simulink model "hyd_hyb_2_sec_con_1"  (Simulink 7.7)
settings: Solver=ode14x  StartTime=0  StopTime=994  FixedStep=0.01  MaxStep=.4  RelTol=1e-8
InitFcn:
  | const_3
values from neighbouring files (symbols this model uses):
  Af = 6.3    [brk_enrg.m]    (also in brk_enrg_1.m)
  BSFC_906_205 = [3.5684 4.3466 5.1668 6.0769 6.988 7.8992 8.8104 9.7336 10.8548 11.9809 13.1112 14.2571 ... (663 elements, 39x17)]    [BSFC_map_906_205.mat]
  Cd = 0.55    [brk_enrg.m]    (also in brk_enrg_1.m)
  den = 1.202    [brk_enrg.m]    (also in brk_enrg_1.m)
  fr = 0.01    [brk_enrg.m]    (also in brk_enrg_1.m)
undefined symbols (not defined in the file or in its folder): clutchRise, down_spd_2, down_spd_3, down_spd_4, down_spd_c, fuel_density, gearshift, I_wheel, Idle_spd_eng_906, M1_hydr, p_v_15, pmax_125, qv_125, Rw, sec_eng_sfc_map, soc_1, soc_2, T_0, T_1, T_2, T_max_906, T_min, t_wait_1, t_wait_2, t_wait_3, TC_spd_ratio_max, torque_convertor, Twait, up_spd_1, up_spd_2, up_spd_3, up_spd_c, v_p_10, v_p_15, v_p_5, veh_spd_0
libraries: fl_lib x43, nesl_utility x30, sdl_lib x14, simulink x5, simulink_need_slupdate x1
(part 3 of 3)

== system hyd_hyb_2_sec_con_1/hydraulic transmission/accumulator/max - min volume estimator/for 10 gal accumulator ==
  min_press(psi) : Inport
  max_press(psi) : Inport  Port=2
  pre_ch_press(psi) : Inport  Port=3
  Action Port : ActionPort  PropagateVarSize=During execution  ActionType=then
  Constant : Constant  Value=152
  Scope : Scope  NumInputPorts=2
      settings: YMin=-5~-5  YMax=5~5  SaveName=ScopeData40
  Scope1 : Scope  NumInputPorts=2
      settings: YMin=-5~-5  YMax=5~5  SaveName=ScopeData41
  in^3 to lit : Gain  Gain=16.387e-3
  in^3 to lit (1) : Gain  Gain=16.387e-3
  rexroth-1 : Lookup_n-D  BreakpointsForDimension1=[1000,1100,1200,1300,1400,1500,1600,1700,1800,1900,2000,2100,2200,2300,2400,2500,2600,2700,2800,2900,3000,3100,3200,3300,3400,3500,3600,3700,3800,3900,4000,4100,4200,4300,4400,4500,4600,4700,4800,4900,5000,5100,5200,5300,5400,5500,5600,5700,5800,5900,6000]  BreakpointsForDimension2=[1000,1400,2000]  Table=v_p_10  InputSameDT=on
  rexroth-10 : Lookup_n-D  BreakpointsForDimension1=[1000,1100,1200,1300,1400,1500,1600,1700,1800,1900,2000,2100,2200,2300,2400,2500,2600,2700,2800,2900,3000,3100,3200,3300,3400,3500,3600,3700,3800,3900,4000,4100,4200,4300,4400,4500,4600,4700,4800,4900,5000,5100,5200,5300,5400,5500,5600,5700,5800,5900,6000]  BreakpointsForDimension2=[1000,1400,2000]  Table=v_p_10  InputSameDT=on
  min_vol(lit) : Outport
  max_vol(lit) : Outport  Port=2
  accum_dry_mass ( kg ) : Outport  Port=3  InitialOutput=[0]
  wires:
  in^3 to lit/1 -> min_vol(lit)/1, Scope1/1
  rexroth-10/1 -> in^3 to lit (1)/1, Scope/2
  rexroth-1/1 -> in^3 to lit/1, Scope/1
  in^3 to lit (1)/1 -> max_vol(lit)/1, Scope1/2
  pre_ch_press(psi)/1 -> rexroth-10/2, rexroth-1/2
  min_press(psi)/1 -> rexroth-1/1
  max_press(psi)/1 -> rexroth-10/1
  Constant/1 -> accum_dry_mass ( kg )/1

== system hyd_hyb_2_sec_con_1/hydraulic transmission/accumulator/max - min volume estimator/for 15 gal accumulator1 ==
  min_press(psi) : Inport
  max_press(psi) : Inport  Port=2
  pre_ch_press(psi) : Inport  Port=3
  Action Port : ActionPort  PropagateVarSize=During execution  ActionType=then
  Constant : Constant  Value=220
  Scope : Scope  NumInputPorts=2
      settings: YMin=-5~-5  YMax=5~5  SaveName=ScopeData38
  Scope1 : Scope  NumInputPorts=2
      settings: YMin=4.74484~24.0403  YMax=4.74484~24.0403  SaveName=ScopeData39
  in^3 to lit : Gain  Gain=16.387e-3
  in^3 to lit (1) : Gain  Gain=16.387e-3
  rexroth-1 : Lookup_n-D  BreakpointsForDimension1=[1000,1100,1200,1300,1400,1500,1600,1700,1800,1900,2000,2100,2200,2300,2400,2500,2600,2700,2800,2900,3000,3100,3200,3300,3400,3500,3600,3700,3800,3900,4000,4100,4200,4300,4400,4500,4600,4700,4800,4900,5000,5100,5200,5300,5400,5500,5600,5700,5800,5900,6000]  BreakpointsForDimension2=[1000,1400,2000]  Table=v_p_15  InputSameDT=on
  rexroth-15 : Lookup_n-D  BreakpointsForDimension1=[1000,1100,1200,1300,1400,1500,1600,1700,1800,1900,2000,2100,2200,2300,2400,2500,2600,2700,2800,2900,3000,3100,3200,3300,3400,3500,3600,3700,3800,3900,4000,4100,4200,4300,4400,4500,4600,4700,4800,4900,5000,5100,5200,5300,5400,5500,5600,5700,5800,5900,6000]  BreakpointsForDimension2=[1000,1400,2000]  Table=v_p_15  InputSameDT=on
  min_vol(lit) : Outport
  max_vol(lit) : Outport  Port=2
  accum_dry_mass ( kg ) : Outport  Port=3  InitialOutput=[0]
  wires:
  in^3 to lit/1 -> min_vol(lit)/1, Scope1/1
  rexroth-1/1 -> in^3 to lit (1)/1, Scope/2
  rexroth-15/1 -> in^3 to lit/1, Scope/1
  in^3 to lit (1)/1 -> max_vol(lit)/1, Scope1/2
  pre_ch_press(psi)/1 -> rexroth-15/2, rexroth-1/2
  min_press(psi)/1 -> rexroth-15/1
  max_press(psi)/1 -> rexroth-1/1
  Constant/1 -> accum_dry_mass ( kg )/1

== system hyd_hyb_2_sec_con_1/hydraulic transmission/accumulator/max - min volume estimator/for 5 gal accumulator ==
  min_press(psi) : Inport
  max_press(psi) : Inport  Port=2
  pre_ch_press(psi) : Inport  Port=3
  Action Port : ActionPort  PropagateVarSize=During execution  ActionType=then
  Constant : Constant  Value=100
  Scope : Scope  NumInputPorts=2
      settings: YMin=-5~-5  YMax=5~5  SaveName=ScopeData27
  Scope1 : Scope  NumInputPorts=2
      settings: YMin=61.8714~626.852  YMax=61.8714~626.852  SaveName=ScopeData28
  in^3 to lit : Gain  Gain=16.387e-3
  in^3 to lit (1) : Gain  Gain=16.387e-3
  rexroth-1 : Lookup_n-D  BreakpointsForDimension1=[1000,1100,1200,1300,1400,1500,1600,1700,1800,1900,2000,2100,2200,2300,2400,2500,2600,2700,2800,2900,3000,3100,3200,3300,3400,3500,3600,3700,3800,3900,4000,4100,4200,4300,4400,4500,4600,4700,4800,4900,5000,5100,5200,5300,5400,5500,5600,5700,5800,5900,6000]  BreakpointsForDimension2=[1000,1400,2000]  Table=v_p_5  InputSameDT=on
  rexroth-5 : Lookup_n-D  BreakpointsForDimension1=[1000,1100,1200,1300,1400,1500,1600,1700,1800,1900,2000,2100,2200,2300,2400,2500,2600,2700,2800,2900,3000,3100,3200,3300,3400,3500,3600,3700,3800,3900,4000,4100,4200,4300,4400,4500,4600,4700,4800,4900,5000,5100,5200,5300,5400,5500,5600,5700,5800,5900,6000]  BreakpointsForDimension2=[1000,1400,2000]  Table=v_p_5  InputSameDT=on
  min_vol(lit) : Outport
  max_vol(lit) : Outport  Port=2
  accum_dry_mass ( kg ) : Outport  Port=3  InitialOutput=[0]
  wires:
  in^3 to lit/1 -> min_vol(lit)/1, Scope/1
  rexroth-1/1 -> in^3 to lit (1)/1, Scope1/2
  rexroth-5/1 -> in^3 to lit/1, Scope1/1
  in^3 to lit (1)/1 -> max_vol(lit)/1, Scope/2
  pre_ch_press(psi)/1 -> rexroth-5/2, rexroth-1/2
  min_press(psi)/1 -> rexroth-5/1
  max_press(psi)/1 -> rexroth-1/1
  Constant/1 -> accum_dry_mass ( kg )/1

== system hyd_hyb_2_sec_con_1/Transmission1/Torque Convertor/main solver/Sensor(TC_in)/Motion sensor ==
  Ideal Rotational Motion Sensor : fl_lib/Mechanical/Mechanical Sensors/Ideal Rotational Motion Sensor  SystemSampleTime=-1  offset=0 rad  w_Log=off  t_Log=off  phi_Log=off  LocalVarNames=|w|t|phi  LocalVarDescs=|w|t|phi  LocalVarLogging=[]
  MRR : fl_lib/Mechanical/Rotational Elements/Mechanical Rotational Reference  SystemSampleTime=-1  t_Log=off  LocalVarNames=|t  LocalVarDescs=|t  LocalVarLogging=[]
  PS-Simulink Converter : nesl_utility/PS-Simulink Converter  SystemSampleTime=-1  PhysicalDomain=network_engine_domain  LeftPortType=input  RightPortType=output  SubClassName=ps_output  Unit=rad/s  AffineConversion=off
  A : PMIOPort  Port=1  Side=Left
  W : Outport
  wires:
  PS-Simulink Converter/1 -> W/1
  connections:
  A/RConn1 -- Ideal Rotational Motion Sensor/LConn1
  Ideal Rotational Motion Sensor/RConn2 -- PS-Simulink Converter/LConn1
  MRR/LConn1 -- Ideal Rotational Motion Sensor/RConn1

== system hyd_hyb_2_sec_con_1/Transmission1/Torque Convertor/main solver/Sensor(TC_in)/Torque sensor ==
  PS2S : nesl_utility/PS-Simulink Converter  SystemSampleTime=-1  PhysicalDomain=network_engine_domain  LeftPortType=input  RightPortType=output  SubClassName=ps_output  Unit=1  AffineConversion=off
  Torque Sensor : fl_lib/Mechanical/Mechanical Sensors/Ideal Torque Sensor  SystemSampleTime=-1  w_Log=off  t_Log=off  LocalVarNames=|w|t  LocalVarDescs=|w|t  LocalVarLogging=[]
  B : PMIOPort  Port=1  Side=Right
  A : PMIOPort  Port=2  Side=Left
  T : Outport
  wires:
  PS2S/1 -> T/1
  connections:
  A/RConn1 -- Torque Sensor/LConn1
  B/RConn1 -- Torque Sensor/RConn1
  Torque Sensor/RConn2 -- PS2S/LConn1

== system hyd_hyb_2_sec_con_1/Transmission1/Torque Convertor/main solver/Sensor(TC_out)/Motion sensor ==
  Ideal Rotational Motion Sensor : fl_lib/Mechanical/Mechanical Sensors/Ideal Rotational Motion Sensor  SystemSampleTime=-1  offset=0 rad  w_Log=off  t_Log=off  phi_Log=off  LocalVarNames=|w|t|phi  LocalVarDescs=|w|t|phi  LocalVarLogging=[]
  MRR : fl_lib/Mechanical/Rotational Elements/Mechanical Rotational Reference  SystemSampleTime=-1  t_Log=off  LocalVarNames=|t  LocalVarDescs=|t  LocalVarLogging=[]
  PS-Simulink Converter : nesl_utility/PS-Simulink Converter  SystemSampleTime=-1  PhysicalDomain=network_engine_domain  LeftPortType=input  RightPortType=output  SubClassName=ps_output  Unit=rad/s  AffineConversion=off
  A : PMIOPort  Port=1  Side=Left
  W : Outport
  wires:
  PS-Simulink Converter/1 -> W/1
  connections:
  MRR/LConn1 -- Ideal Rotational Motion Sensor/RConn1
  Ideal Rotational Motion Sensor/RConn2 -- PS-Simulink Converter/LConn1
  A/RConn1 -- Ideal Rotational Motion Sensor/LConn1

== system hyd_hyb_2_sec_con_1/Transmission1/Torque Convertor/main solver/Sensor(TC_out)/Torque sensor ==
  PS2S : nesl_utility/PS-Simulink Converter  SystemSampleTime=-1  PhysicalDomain=network_engine_domain  LeftPortType=input  RightPortType=output  SubClassName=ps_output  Unit=1  AffineConversion=off
  Torque Sensor : fl_lib/Mechanical/Mechanical Sensors/Ideal Torque Sensor  SystemSampleTime=-1  w_Log=off  t_Log=off  LocalVarNames=|w|t  LocalVarDescs=|w|t  LocalVarLogging=[]
  B : PMIOPort  Port=1  Side=Right
  A : PMIOPort  Port=2  Side=Left
  T : Outport
  wires:
  PS2S/1 -> T/1
  connections:
  Torque Sensor/RConn2 -- PS2S/LConn1
  B/RConn1 -- Torque Sensor/RConn1
  A/RConn1 -- Torque Sensor/LConn1

== system hyd_hyb_2_sec_con_1/Transmission1/gear box/gear box/Clutch Control/Enabled Subsystem1 ==
  Enable : EnablePort  StatesWhenEnabling=reset  PropagateVarSize=During execution
  Clutch A Actuator : TransferFcn  Numerator=[1/clutchRise]  Denominator=[1 1/clutchRise]
  engage : Constant
  clutch release : Outport  OutputWhenDisabled=reset  InitialOutput=[0]
  wires:
  engage/1 -> Clutch A Actuator/1
  Clutch A Actuator/1 -> clutch release/1

== system hyd_hyb_2_sec_con_1/Transmission1/gear box/gear box/Clutch Control/Enabled Subsystem2 ==
  Enable : EnablePort  StatesWhenEnabling=reset  PropagateVarSize=During execution
  Clutch A Actuator : TransferFcn  Numerator=[1/clutchRise]  Denominator=[1 1/clutchRise]
  engage : Constant
  clutch release : Outport  OutputWhenDisabled=reset  InitialOutput=[0]
  wires:
  Clutch A Actuator/1 -> clutch release/1
  engage/1 -> Clutch A Actuator/1

== system hyd_hyb_2_sec_con_1/Transmission1/gear box/gear box/Clutch Control/Enabled Subsystem3 ==
  Enable : EnablePort  StatesWhenEnabling=reset  PropagateVarSize=During execution
  Clutch A Actuator : TransferFcn  Numerator=[1/clutchRise]  Denominator=[1 1/clutchRise]
  engage : Constant
  clutch release : Outport  OutputWhenDisabled=reset  InitialOutput=[0]
  wires:
  engage/1 -> Clutch A Actuator/1
  Clutch A Actuator/1 -> clutch release/1

== system hyd_hyb_2_sec_con_1/Transmission1/gear box/gear box/Clutch Control/Enabled Subsystem4 ==
  Enable : EnablePort  StatesWhenEnabling=reset  PropagateVarSize=During execution
  Clutch A Actuator : TransferFcn  Numerator=[1/clutchRise]  Denominator=[1 1/clutchRise]
  engage : Constant
  clutch release : Outport  OutputWhenDisabled=reset  InitialOutput=[0]
  wires:
  Clutch A Actuator/1 -> clutch release/1
  engage/1 -> Clutch A Actuator/1

== stateflow chart driver/Chart ==
  state transmission state control [group]
    state Drive
      during: s=1;
    state Neutral
      during: s=0;
    (default) -> Neutral
    Neutral -> Drive : [cyc> 0]
    Drive -> Neutral : after(1,sec)[cyc== 0]
  data: cyc input double; speed input double; s output double

== stateflow chart Transmission1/transmission control/Chart1 ==
  state fourth
    entry: gear = 4;
  state third
    entry: gear = 3;
  state second
    entry: gear = 2;
  state first
    entry: TC=1;
  state firstc
    entry: gear=1;
    entry: TC=0;
  second -> third [order 1] : after(Twait,tick)
      | [speed >= up_spd_2]
  first -> second [order 1] : after(Twait,tick)
      | [speed >= up_spd_1]
  third -> fourth [order 1] : after(Twait,tick)
      | [speed >= up_spd_3]
  firstc -> first : after(Twait,tick)
      | [speed >=up_spd_c]
  (default) -> firstc
  third -> second [order 2] : after(Twait,tick)
      | [speed < down_spd_3]
  fourth -> third : after(Twait,tick)
      | [speed < down_spd_4]
  first -> firstc [order 2] : after(Twait,tick)
      | [speed < down_spd_c]
  second -> first [order 2] : after(Twait,tick)
      | [speed < down_spd_2]
  data: speed input double; gear output double; TC output double; down_spd_4 parameter double; down_spd_2 parameter double; down_spd_3 parameter double; up_spd_1 parameter double; up_spd_2 parameter double; up_spd_3 parameter double; down_spd_c parameter double; up_spd_c parameter double; Twait parameter double

== stateflow chart controller/control strategy - acceleration torque estimator/control strategy ==
  state state1
    during: T_pm=min(1.8*delta_p,T_acc);T_eng =T_acc-T_pm;u=1;
  state state2
    during: u=2;
    state state2
      during: T_eng=T_acc;T_pm=0;
    state state3
      during: T_eng=T_2;T_pm=T_acc-T_eng;
    state state1
      during:T_pm=(1.8*delta_p)*((T_1-T_acc)/100);
      T_eng=T_acc-T_pm;
    (default) -> state2.state1
    state2.state3 -> state2.state2 : [T_acc<=T_2]
    state2.state2 -> state2.state1 [order 2] : [T_acc<=T_1]
    state2.state2 -> state2.state3 [order 1] : [T_acc>T_2]
    state2.state1 -> state2.state2 : [T_acc>T_1]
  state state3
    during: u=3;T_eng=T_acc;T_pm=0;
  (default) -> state1
  state1 -> state2 [order 2] : [veh_spd>veh_spd_0 && T_acc>=T_0 && soc>soc_1]
  state2 -> state3 [order 1] : [soc<=soc_1]
  state3 -> state2 [order 2] : [soc>=soc_2 && T_acc>T_0]
  state3 -> state1 [order 1] : [soc>=soc_2 && T_acc<T_0]
  state1 -> state3 [order 1] : [soc<=soc_1]
  state2 -> state1 [order 2] : [soc>=soc_1 && T_acc<T_0]
  data: T_acc input double; soc input double; T_eng output double; T_pm output double; x input double; veh_spd input double; y input double; T_0 parameter double; T_1 parameter double; soc_1 parameter double; soc_2 parameter double; t_wait_1 parameter double; t_wait_2 parameter double; t_wait_3 parameter double; veh_spd_0 parameter double; u output double; delta_p input double; T_2 parameter double

== stateflow chart hydraulic transmission/PM_hydraulic_machine /qv - pmax evaluation/Chart ==
  state state1
    during: u1=1;
  state state2
    during: u1=0;
  (default) -> state1
  state1 -> state2 : [soc <= soc_min]
  state2 -> state1 : [soc > 50]
  data: soc input double; soc_min input double; u1 output double
